simulink model "Real_Acrobot_Simulation"  (R2022b)
settings: Solver=ode23t  StartTime=0.0  StopTime=35  FixedStep=0.0002  MaxStep=1.6  RelTol=1e-4
values from neighbouring files (symbols this model uses):
  g = 9.81    [linearizalas.m]    (also in real_parameters.m)
  K = inv(R+B_d'*P*B_d)*B_d'*P*A_d    [DLQR.m]    (also in Main.m = LQR_function(A, B))
  l1 = 0.4    [real_parameters.m]
  m_weight = 0.086    [real_parameters.m]
  Q0 = [0.1 0 0 0]    [real_parameters.m]
undefined symbols (not defined in the file or in its folder): X, Y, Z
libraries: sm_lib x44, nesl_utility x22, fl_lib x15, simulink_extras x4, ee_lib x2, hdlsllib x1, eeQuadratureDecoder x1, slpidlib x1, simulink x1
(part 2 of 2)

== system Real_Acrobot_Simulation/Acrobot modelling/Joint 1/Encoder ==
  Electrical Reference : fl_lib/Electrical/Electrical Elements/Electrical Reference
  Incremental Shaft Encoder : ee_lib/Sensors & Transducers/Incremental Shaft Encoder  NPulse=600  Vm=5 V  angle0=0 deg
      settings: InternalSimscapePortConfiguration="{\"Bottom\":[],\"Left\":[{\"id\":\"R\",\"label\":\"R\",\"type\":\"foundation.mechanical.rotational.rotational\"},{\"id\":\"C\",\"label\":\"C\",\"type\":\"foundation.mechanical.rotational.rotational\"}],\"Right\":[{\"id\":\"A\",\"label\":\"A\",\"type\":\"foundation.electrical.electrical\"},{\"id\":\"B\",\"label\":\"B\",\"type\":\"foundation.electrical.electrical\"},{\"id\":\"Z\",\"label\":\"Z\",\"type\":\"foundation.electrical.electrical\"},{\"id\":\"GND\",\"label\":\"REF\",\"type\":\"foundation.electrical.electrical\"}],\"Top\":[]}"
  Mechanical Rotational Reference1 : fl_lib/Mechanical/Rotational Elements/Mechanical Rotational Reference
  PS-Simulink Converter : nesl_utility/PS-Simulink Converter  PhysicalDomain=network_engine_domain  SubClassName=ps_output  LeftPortType=input  RightPortType=output  PseudoPeriodic=off  Frequencies=[]  VectorFormat=1-D array  Unit=inherit  AffineConversion=off
  PS-Simulink Converter4 : nesl_utility/PS-Simulink Converter  PhysicalDomain=network_engine_domain  SubClassName=ps_output  LeftPortType=input  RightPortType=output  PseudoPeriodic=off  Frequencies=[]  VectorFormat=1-D array  Unit=inherit  AffineConversion=off
  Rotational Multibody Interface : fl_lib/Mechanical/Multibody Interfaces/Rotational Multibody Interface
  Voltage Sensor4 : fl_lib/Electrical/Electrical Sensors/Voltage Sensor
  Voltage Sensor5 : fl_lib/Electrical/Electrical Sensors/Voltage Sensor
  dq1 : PMIOPort  Side=Left
  B : Outport
  A : Outport  Port=2
  wires:
  PS-Simulink Converter/1 -> A/1
  PS-Simulink Converter4/1 -> B/1
  connections:
  Incremental Shaft Encoder/LConn1 -- Rotational Multibody Interface/RConn2
  Electrical Reference/LConn1 -- Incremental Shaft Encoder/RConn4 -- Voltage Sensor5/RConn2 -- Voltage Sensor4/RConn2
  dq1/RConn1 -- Rotational Multibody Interface/RConn1
  Mechanical Rotational Reference1/LConn1 -- Rotational Multibody Interface/LConn2 -- Incremental Shaft Encoder/LConn2
  Voltage Sensor4/LConn1 -- Incremental Shaft Encoder/RConn2
  Voltage Sensor5/LConn1 -- Incremental Shaft Encoder/RConn1
  Voltage Sensor4/RConn1 -- PS-Simulink Converter4/LConn1
  Voltage Sensor5/RConn1 -- PS-Simulink Converter/LConn1

== system Real_Acrobot_Simulation/Acrobot modelling/Joint 1/Revolute Join1 ==
  Joint1 : sm_lib/Joints/Revolute Joint  JointMode=Normal  SenseConstraintForce=off  SenseConstraintForceX=off  SenseConstraintForceY=off  SenseConstraintForceZ=off  SenseConstraintTorque=off  SenseConstraintTorqueX=off  SenseConstraintTorqueY=off  SenseConstraintTorqueZ=off  SenseTotalForce=off  SenseTotalForceX=off  SenseTotalForceY=off  SenseTotalForceZ=off  SenseTotalTorque=off  SenseTotalTorqueX=off  SenseTotalTorqueY=off  SenseTotalTorqueZ=off  CompositeWrenchDir=FollowerOnBase  CompositeWrenchFrame=BaseFrame  EquilibriumPosition=0  EquilibriumPositionUnits=deg  SpringStiffness=0  SpringStiffnessUnits=N*m/deg  DampingCoefficient=0.002  DampingCoefficientUnits=N*m/(rad/s)  TorqueActuationMode=NoTorque  MotionActuationMode=ComputedMotion  SensePosition=on  SenseVelocity=on  SenseAcceleration=off  SenseTorqueForce=off  SenseLowerLimitTorqueForce=off  SenseUpperLimitTorqueForce=off  LowerLimitSpecify=off  LowerLimitBound=-90  LowerLimitBoundUnits=deg  LowerLimitStiffness=1e4  LowerLimitStiffnessUnits=N*m/deg  LowerLimitDamping=10  LowerLimitDampingUnits=N*m/(deg/s)  LowerLimitTransitionRegionWidth=0.1  LowerLimitTransitionRegionWidthUnits=deg  UpperLimitSpecify=off  UpperLimitBound=90  UpperLimitBoundUnits=deg  UpperLimitStiffness=1e4  UpperLimitStiffnessUnits=N*m/deg  UpperLimitDamping=10  UpperLimitDampingUnits=N*m/(deg/s)  UpperLimitTransitionRegionWidth=0.1  UpperLimitTransitionRegionWidthUnits=deg  PositionTargetSpecify=on  PositionTargetPriority=High  PositionTargetValue=Q0(1)  PositionTargetValueUnits=rad  VelocityTargetSpecify=on  VelocityTargetPriority=High  VelocityTargetValue=Q0(2)  VelocityTargetValueUnits=rad/s
  PS-Simulink Converter2 : nesl_utility/PS-Simulink Converter  PhysicalDomain=network_engine_domain  SubClassName=ps_output  LeftPortType=input  RightPortType=output  PseudoPeriodic=off  Frequencies=[]  VectorFormat=1-D array  Unit=inherit  AffineConversion=off
  PS-Simulink Converter3 : nesl_utility/PS-Simulink Converter  PhysicalDomain=network_engine_domain  SubClassName=ps_output  LeftPortType=input  RightPortType=output  PseudoPeriodic=off  Frequencies=[]  VectorFormat=1-D array  Unit=inherit  AffineConversion=off
  Trans Z1 : sm_lib/Frames and Transforms/Rigid Transform  TranslationMethod=StandardAxis  TranslationStandardOffset=2  TranslationLengthUnit=cm  TranslationStandardAxis=+Z  TranslationCartesianOffset=[0 0 0]  TranslationROffset=0  TranslationROffsetUnits=m  TranslationZOffset=0  TranslationZOffsetUnits=m  TranslationThetaOffset=0  TranslationThetaOffsetUnits=deg  RotationMethod=None  RotationAngleUnits=deg  RotationStandardAxis=+X  RotationAngle=90  RotationArbitraryAxis=[0 0 1]  FollAlignAxisA=+X  BaseAlignAxisA=+Y  FollAlignAxisB=+Y  BaseAlignAxisB=+Z  RotationSequenceAxes=FollowerAxes  RotationSequence=XYX  RotationSequenceAngles=[0 0 0]  RotationSequenceAnglesUnits=deg  RotationMatrix=[1 0 0; 0 1 0; 0 0 1]  Quaternion=[1 0 0 0]
  " In" : PMIOPort  Side=Left
  dq1_mech : PMIOPort  Port=2  Side=Right
  Out : PMIOPort  Port=3  Side=Right
  q1 : Outport
  dq1 : Outport  Port=2
  wires:
  PS-Simulink Converter2/1 -> q1/1
  PS-Simulink Converter3/1 -> dq1/1
  connections:
  Trans Z1/RConn1 -- Joint1/LConn1
  Joint1/RConn1 -- Out/RConn1
  Trans Z1/LConn1 -- " In"/RConn1
  Joint1/RConn3 -- PS-Simulink Converter3/LConn1 -- dq1_mech/RConn1
  PS-Simulink Converter2/LConn1 -- Joint1/RConn2

== system Real_Acrobot_Simulation/Acrobot modelling/Joint 1/Wrap Angle ==
  In1 : Inport
  Add1 : Sum  Inputs=+-
  Bias : Bias  Bias=pi  SaturateOnIntegerOverflow=off
  Constant : Constant  Value=2*pi
  Constant2 : Constant  Value=2*pi
  Divide : Product  Inputs=*/
  Floor : Rounding
  Product : Product  Inputs=**
  q1 : Outport
  wires:
  Constant/1 -> Divide/2
  In1/1 -> Bias/1, Add1/1
  Divide/1 -> Floor/1
  Floor/1 -> Product/1
  Constant2/1 -> Product/2
  Product/1 -> Add1/2
  Add1/1 -> q1/1
  Bias/1 -> Divide/1

== system Real_Acrobot_Simulation/Acrobot modelling/Joint 1/Wrap Angle pi-pi ==
  In1 : Inport
  Add1 : Sum  Inputs=+-
  Bias : Bias  Bias=pi  SaturateOnIntegerOverflow=off
  Constant : Constant  Value=2*pi
  Constant2 : Constant  Value=2*pi
  Divide : Product  Inputs=*/
  Floor : Rounding
  Product : Product  Inputs=**
  q1 : Outport
  wires:
  Constant/1 -> Divide/2
  In1/1 -> Bias/1, Add1/1
  Divide/1 -> Floor/1
  Floor/1 -> Product/1
  Constant2/1 -> Product/2
  Product/1 -> Add1/2
  Add1/1 -> q1/1
  Bias/1 -> Divide/1

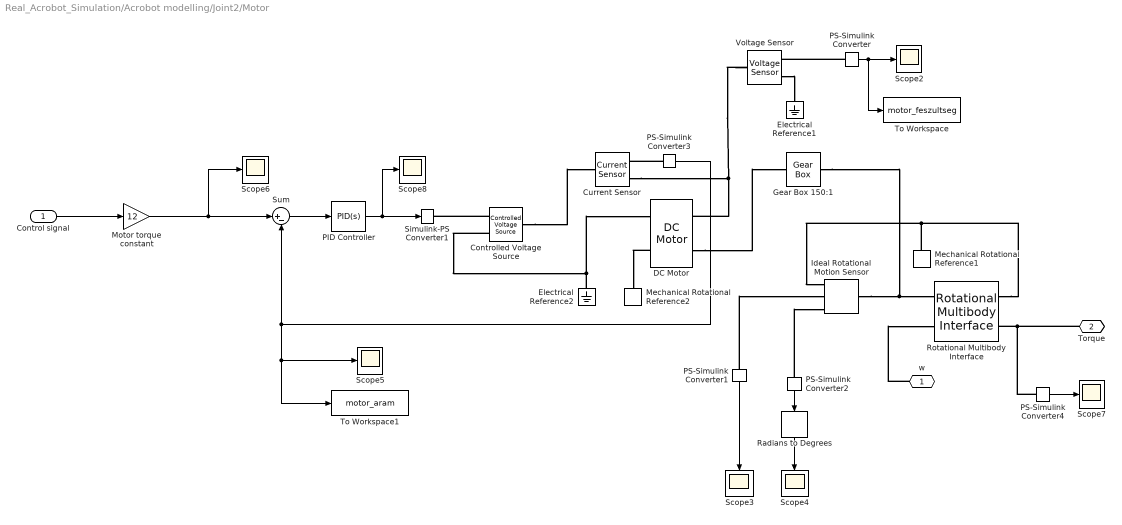
== system Real_Acrobot_Simulation/Acrobot modelling/Joint2/Motor ==
  Control signal : Inport
  Controlled Voltage Source : fl_lib/Electrical/Electrical Sources/Controlled Voltage Source
  Current Sensor : fl_lib/Electrical/Electrical Sensors/Current Sensor
  DC Motor : ee_lib/Electromechanical/Brushed Motors/DC Motor  field_option=ee.enum.field_option.pm  Rf=100 Ohm  Lf=1 H  Laf=0.15 H  If0=0 A  parameterization=ee.enum.dcparam_option.circuit_param  Ra=3.9 Ohm  La=12e-6 H  emf_or_torque=ee.enum.emf_or_torque.kv  Kv=0.072e-3 V/rpm  Ki=6.876e-4 N*m/A  T_stall=0.24e-3 N*m  w_max=19100 rpm  w_rated=15000 rpm  P_rated=0.08 W  V_rated=1.5 V  lam_param=ee.enum.lam_param.damping  i_noload=0 A  V_i_noload=1.5 V  J=0.01 cm^2*g  lam=0 N*m*s/rad  speed0=0 rpm  enable_fault_armature=simscape.enum.onoff.off  rev_faulted=1 / 3  G_faulted_armature=1e-5 S  fault_trigger_armature=ee.enum.faults.faultTrigger.temporal  t_fault_armature=1 s  max_permissible_current_armature=inf A  t_fail_on_current_armature=1 s  enable_fault_field=simscape.enum.onoff.off  G_faulted_field=1e-5 S  fault_trigger_field=ee.enum.faults.faultTrigger.temporal  t_fault_field=1 s  max_permissible_current_field=inf A  t_fail_on_current_field=1 s  fault_action=simscape.enum.assert.action.none  alpha=3.93e-3 1/K  Tmeas=25 degC  thermal_mass=100 J/K  initial_temperature=25 degC
  Electrical Reference1 : fl_lib/Electrical/Electrical Elements/Electrical Reference
  Electrical Reference2 : fl_lib/Electrical/Electrical Elements/Electrical Reference
  Gear Box 150:1 : fl_lib/Mechanical/Mechanisms/Gear Box  ratio=150  t_in_specify=off  t_in_priority=None  t_in=0 N*m  t_in_nominal_specify=off  t_in_nominal_unit=N*m  t_in_nominal_value=1  t_out_specify=off  t_out_priority=None  t_out=0 N*m  t_out_nominal_specify=off  t_out_nominal_unit=N*m  t_out_nominal_value=1
  Ideal Rotational Motion Sensor : fl_lib/Mechanical/Mechanical Sensors/Ideal Rotational Motion Sensor  reference=foundation.enum.MeasurementReference.difference  acceleration_port=false  velocity_port=true  position_port=true  wrap_angle=false  offset=0 rad
  Mechanical Rotational Reference1 : fl_lib/Mechanical/Rotational Elements/Mechanical Rotational Reference
  Mechanical Rotational Reference2 : fl_lib/Mechanical/Rotational Elements/Mechanical Rotational Reference
  Motor torque constant : Gain  Gain=12
  PID Controller : slpidlib/PID Controller  Controller=PID  Form=Parallel  TimeDomain=Continuous-time  UseExternalTs=off  SampleTime=-1  IntegratorMethod=Forward Euler  FilterMethod=Forward Euler  ControllerParametersSource=internal  P=10  I=0.1  UseKiTs=off  D=0.5  N=100  UseFilter=on  TunerSelectOption=Transfer Function Based (PID Tuner App)  InitialConditionSource=internal  InitialConditionForIntegrator=0  InitialConditionForFilter=0  DifferentiatorICPrevScaledInput=0  ExternalReset=none  TrackingMode=off  Kt=1  LimitOutput=off  SatLimitsSource=internal  UpperSaturationLimit=inf  LowerSaturationLimit=-inf  LinearizeAsGain=on  AntiWindupMode=none  Kb=1  LimitIntegrator=off  UpperIntegratorSaturationLimit=inf  LowerIntegratorSaturationLimit=-inf  POutMin=[]  POutMax=[]  IOutMin=[]  IOutMax=[]  DOutMin=[]  DOutMax=[]  NOutMin=[]  NOutMax=[]  SumOutMin=[]  SumOutMax=[]  SaturationOutMin=[]  SaturationOutMax=[]  PParamMin=[]  PParamMax=[]  IParamMin=[]  IParamMax=[]  DParamMin=[]  DParamMax=[]  NParamMin=[]  NParamMax=[]  KbParamMin=[]  KbParamMax=[]  KtParamMin=[]  KtParamMax=[]  KbOutMin=[]  KbOutMax=[]  KtOutMin=[]  KtOutMax=[]  IntegratorOutMin=[]  IntegratorOutMax=[]  FilterOutMin=[]  FilterOutMax=[]  SumI1OutMin=[]  SumI1OutMax=[]  SumI2OutMin=[]  SumI2OutMax=[]  SumI3OutMin=[]  SumI3OutMax=[]  SumI4OutMin=[]  SumI4OutMax=[]  SumDOutMin=[]  SumDOutMax=[]  DifferentiatorOutMin=[]  DifferentiatorOutMax=[]  FilterDiffOutCoefMin=[]  FilterDiffOutCoefMax=[]  ReciprocalOutMin=[]  ReciprocalOutMax=[]  SumDenOutMin=[]  SumDenOutMax=[]  SumNumOutMin=[]  SumNumOutMax=[]  DivideOutMin=[]  DivideOutMax=[]  UdiffTsProdOutMin=[]  UdiffTsProdOutMax=[]  NTsProdOutMin=[]  NTsProdOutMax=[]  UintegralTsProdOutMin=[]  UintegralTsProdOutMax=[]  UngainTsProdOutMin=[]  UngainTsProdOutMax=[]  ClampingZeroOutDataTypeStr=Inherit: Inherit via back propagation  ClampingZeroOutMin=[]  ClampingZeroOutMax=[]  FilterDenConstantOutDataTypeStr=Inherit: Inherit via back propagation  FilterDenConstantOutMin=[]  FilterDenConstantOutMax=[]  PCopyOutDataTypeStr=Inherit: Inherit via back propagation  PCopyOutMin=[]  PCopyOutMax=[]  NCopyOutDataTypeStr=Inherit: Inherit via back propagation  NCopyOutMin=[]  NCopyOutMax=[]  IntegratorContinuousStateAttributes=''  IntegratorStateMustResolveToSignalObject=off  IntegratorRTWStateStorageClass=Auto  FilterContinuousStateAttributes=''  FilterStateMustResolveToSignalObject=off  FilterRTWStateStorageClass=Auto  ParallelPVariant=InternalParameters  IdealPVariant=Disabled  IVariant=InternalParameters  DVariant=InternalParameters  IntegratorVariant=Continuous  SatVariant=Disabled  AWVariant=Passthrough  PCopyVariant=Disabled  TRVariant=Disabled  FdbkBlocksVariant=Forward  IdealPFdbkVariant=Disabled  SatFdbkVariant=Disabled  DerivativeFilterVariant=ContFilter  NVariant=InternalParameters  NCopyVariant=Disabled  FilterICVariant=InternalICsFilter  IntegratorICVariant=InternalICs  ExternalResetVariant=Disabled  TRSumVariant=Passthrough  SumFdbkVariant=Disabled  SumVariant=Sum_PID  TsampFilterVariant=InternalTs  TsampNgainVariant=Passthrough  TsampIntegralVariant=Passthrough  ExternalSaturationOutDataTypeStr=Inherit: Same as second input
  PS-Simulink Converter{,1..2,4} (4 alike) : nesl_utility/PS-Simulink Converter  PhysicalDomain=network_engine_domain  SubClassName=ps_output  LeftPortType=input  RightPortType=output  PseudoPeriodic=off  Frequencies=[]  VectorFormat=1-D array  Unit=inherit  AffineConversion=off
  PS-Simulink Converter3 : nesl_utility/PS-Simulink Converter  PhysicalDomain=network_engine_domain  SubClassName=ps_output  LeftPortType=input  RightPortType=output  PseudoPeriodic=off  Frequencies=[]  VectorFormat=inherit  Unit=inherit  AffineConversion=off
  Radians to Degrees : simulink_extras/Transformations/Radians to Degrees
  Rotational Multibody Interface : fl_lib/Mechanical/Multibody Interfaces/Rotational Multibody Interface
  Scope{2..8} (7 alike) : Scope
  Simulink-PS Converter1 : nesl_utility/Simulink-PS Converter  PhysicalDomain=network_engine_domain  SubClassName=ps_input  LeftPortType=input  RightPortType=output  PseudoPeriodic=off  Frequencies=[]  NoiseDistribution=none  NoiseParameters=[]  Unit=1  AffineConversion=off  FilteringAndDerivatives=provide  SimscapeFilterOrder=1  InputFilterTimeConstant=0.001  UdotUserProvided=0
  Sum : Sum  Inputs=|+-
  To Workspace : ToWorkspace  VariableName=motor_feszultseg  SaveFormat=Timeseries  SampleTime=-1
  To Workspace1 : ToWorkspace  VariableName=motor_aram  SaveFormat=Timeseries  SampleTime=-1
  Voltage Sensor : fl_lib/Electrical/Electrical Sensors/Voltage Sensor
  w : PMIOPort  Side=Left
  Torque : PMIOPort  Port=2  Side=Right
  wires:
  PS-Simulink Converter/1 -> To Workspace/1, Scope2/1
  PS-Simulink Converter2/1 -> Radians to Degrees/1
  Radians to Degrees/1 -> Scope4/1
  PS-Simulink Converter1/1 -> Scope3/1
  Control signal/1 -> Motor torque constant/1
  Motor torque constant/1 -> Scope6/1, Sum/1
  PS-Simulink Converter3/1 -> Sum/2, Scope5/1, To Workspace1/1
  PS-Simulink Converter4/1 -> Scope7/1
  Sum/1 -> PID Controller/1
  PID Controller/1 -> Simulink-PS Converter1/1, Scope8/1
  connections:
  PS-Simulink Converter/LConn1 -- Voltage Sensor/RConn1
  Mechanical Rotational Reference1/LConn1 -- Ideal Rotational Motion Sensor/RConn1 -- Rotational Multibody Interface/LConn2
  Ideal Rotational Motion Sensor/LConn1 -- Gear Box 150:1/RConn1 -- Rotational Multibody Interface/RConn2
  PS-Simulink Converter1/LConn1 -- Ideal Rotational Motion Sensor/RConn2
  PS-Simulink Converter2/LConn1 -- Ideal Rotational Motion Sensor/RConn3
  Voltage Sensor/RConn2 -- Electrical Reference1/LConn1
  Torque/RConn1 -- PS-Simulink Converter4/LConn1 -- Rotational Multibody Interface/LConn1
  DC Motor/RConn2 -- Mechanical Rotational Reference2/LConn1
  PS-Simulink Converter3/LConn1 -- Current Sensor/RConn1
  Electrical Reference2/LConn1 -- DC Motor/RConn1 -- Controlled Voltage Source/RConn2
  Current Sensor/RConn2 -- Voltage Sensor/LConn1 -- DC Motor/LConn1
  DC Motor/LConn2 -- Gear Box 150:1/LConn1
  w/RConn1 -- Rotational Multibody Interface/RConn1
  Controlled Voltage Source/LConn1 -- Current Sensor/LConn1
  Controlled Voltage Source/RConn1 -- Simulink-PS Converter1/RConn1

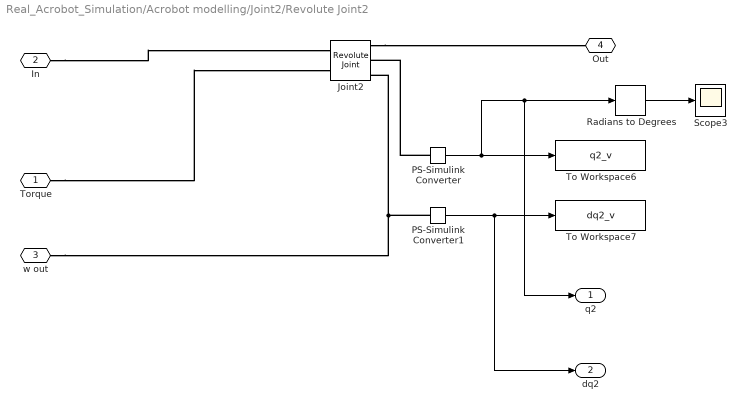
== system Real_Acrobot_Simulation/Acrobot modelling/Joint2/Revolute Joint2 ==
  Joint2 : sm_lib/Joints/Revolute Joint  JointMode=Normal  SenseConstraintForce=off  SenseConstraintForceX=off  SenseConstraintForceY=off  SenseConstraintForceZ=off  SenseConstraintTorque=off  SenseConstraintTorqueX=off  SenseConstraintTorqueY=off  SenseConstraintTorqueZ=off  SenseTotalForce=off  SenseTotalForceX=off  SenseTotalForceY=off  SenseTotalForceZ=off  SenseTotalTorque=off  SenseTotalTorqueX=off  SenseTotalTorqueY=off  SenseTotalTorqueZ=off  CompositeWrenchDir=FollowerOnBase  CompositeWrenchFrame=BaseFrame  EquilibriumPosition=0  EquilibriumPositionUnits=deg  SpringStiffness=0  SpringStiffnessUnits=N*m/deg  DampingCoefficient=0  DampingCoefficientUnits=N*m/(deg/s)  TorqueActuationMode=InputTorque  MotionActuationMode=ComputedMotion  SensePosition=on  SenseVelocity=on  SenseAcceleration=off  SenseTorqueForce=off  SenseLowerLimitTorqueForce=off  SenseUpperLimitTorqueForce=off  LowerLimitSpecify=on  LowerLimitBound=-90  LowerLimitBoundUnits=deg  LowerLimitStiffness=1e4  LowerLimitStiffnessUnits=N*m/deg  LowerLimitDamping=10  LowerLimitDampingUnits=N*m/(deg/s)  LowerLimitTransitionRegionWidth=0.1  LowerLimitTransitionRegionWidthUnits=deg  UpperLimitSpecify=on  UpperLimitBound=90  UpperLimitBoundUnits=deg  UpperLimitStiffness=1e4  UpperLimitStiffnessUnits=N*m/deg  UpperLimitDamping=10  UpperLimitDampingUnits=N*m/(deg/s)  UpperLimitTransitionRegionWidth=0.1  UpperLimitTransitionRegionWidthUnits=deg  PositionTargetSpecify=on  PositionTargetPriority=High  PositionTargetValue=Q0(3)  PositionTargetValueUnits=rad  VelocityTargetSpecify=on  VelocityTargetPriority=High  VelocityTargetValue=Q0(4)  VelocityTargetValueUnits=rad/s
  PS-Simulink Converter : nesl_utility/PS-Simulink Converter  PhysicalDomain=network_engine_domain  SubClassName=ps_output  LeftPortType=input  RightPortType=output  PseudoPeriodic=off  Frequencies=[]  VectorFormat=1-D array  Unit=inherit  AffineConversion=off
  PS-Simulink Converter1 : nesl_utility/PS-Simulink Converter  PhysicalDomain=network_engine_domain  SubClassName=ps_output  LeftPortType=input  RightPortType=output  PseudoPeriodic=off  Frequencies=[]  VectorFormat=1-D array  Unit=inherit  AffineConversion=off
  Radians to Degrees : simulink_extras/Transformations/Radians to Degrees
  Scope3 : Scope
  To Workspace6 : ToWorkspace  VariableName=q2_v  SaveFormat=Timeseries  SampleTime=-1
  To Workspace7 : ToWorkspace  VariableName=dq2_v  SaveFormat=Timeseries  SampleTime=-1
  Torque : PMIOPort  Side=Left
  In : PMIOPort  Port=2  Side=Left
  w out : PMIOPort  Port=3  Side=Right
  Out : PMIOPort  Port=4  Side=Right
  q2 : Outport
  dq2 : Outport  Port=2
  wires:
  PS-Simulink Converter1/1 -> dq2/1, To Workspace7/1
  PS-Simulink Converter/1 -> Radians to Degrees/1, q2/1, To Workspace6/1
  Radians to Degrees/1 -> Scope3/1
  connections:
  PS-Simulink Converter/LConn1 -- Joint2/RConn2
  PS-Simulink Converter1/LConn1 -- Joint2/RConn3 -- w out/RConn1
  In/RConn1 -- Joint2/LConn1
  Joint2/RConn1 -- Out/RConn1
  Torque/RConn1 -- Joint2/LConn2

== system Real_Acrobot_Simulation/Acrobot modelling/Controller/Controller/LQR Control ==
  note: Balancing - linearizalt rendszerre
  note: -pi eltolas
      | A linearizalt szabalyozashoz csak
      | itt meg akar modulot probalgatni
  note: q1 q2 dq1 dq2
  note: q1 q2 dq1 dq2
  States : Inport
  Bias : Bias  Bias=-pi  SaturateOnIntegerOverflow=off
  Demux1 : Demux
  Gain : Gain  Gain=-K  Multiplication=Matrix(K*u)
  Mux1 : Mux
  Scope1 : Scope
  Scope2 : Scope
  Wrap Angle pi-pi : Subsystem
  Control signal : Outport
  wires:
  Mux1/1 -> Gain/1, Scope1/1
  States/1 -> Demux1/1
  Demux1/1 -> Bias/1
  Demux1/4 -> Mux1/4
  Demux1/2 -> Mux1/2
  Demux1/3 -> Mux1/3
  Bias/1 -> Wrap Angle pi-pi/1(In1)
  Wrap Angle pi-pi/1(q1) -> Mux1/1
  Gain/1 -> Control signal/1, Scope2/1

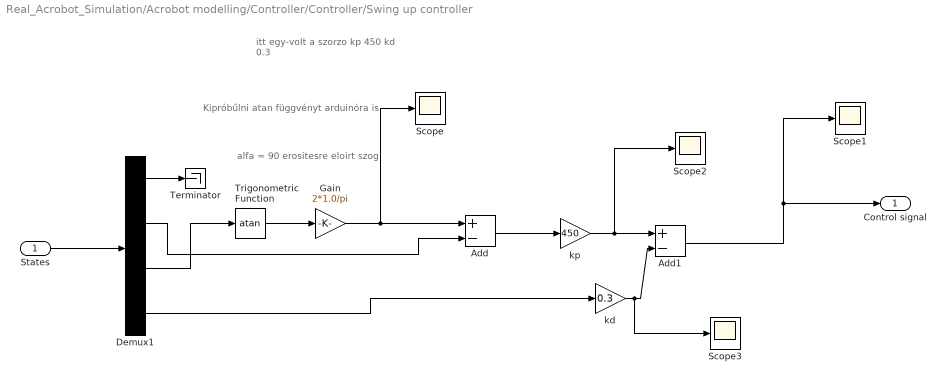
== system Real_Acrobot_Simulation/Acrobot modelling/Controller/Controller/Swing up controller ==
  note: itt egy-volt a szorzo
      | kp 450
      | kd 0.3
  note: Kipróbűlni atan függvényt arduinóra is
  note: alfa = 90 erositesre eloirt szog
  States : Inport
  Add : Sum  Inputs=+-
  Add1 : Sum  Inputs=+-
  Demux1 : Demux
  Gain : Gain  Gain=2*1.0/pi
  Scope{,1..3} (4 alike) : Scope
  Terminator : Terminator
  Trigonometric Function : Trigonometry  Operator=atan
  kd : Gain  Gain=0.3
  kp : Gain  Gain=450
  Control signal : Outport
  wires:
  States/1 -> Demux1/1
  Trigonometric Function/1 -> Gain/1
  Gain/1 -> Add/1, Scope/1
  kd/1 -> Scope3/1, Add1/2
  Demux1/4 -> kd/1
  Add1/1 -> Scope1/1, Control signal/1
  Demux1/1 -> Terminator/1
  Demux1/3 -> Trigonometric Function/1
  Demux1/2 -> Add/2
  Add/1 -> kp/1
  kp/1 -> Add1/1, Scope2/1

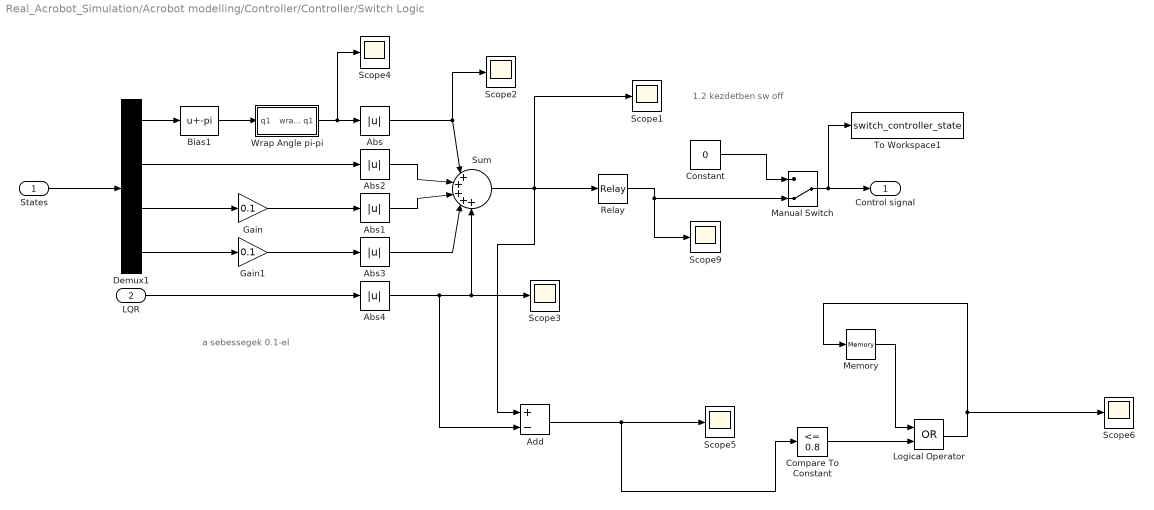
== system Real_Acrobot_Simulation/Acrobot modelling/Controller/Controller/Switch Logic ==
  note: a sebessegek 0.1-el
  note: 1.2 kezdetben sw off
  States : Inport
  LQR : Inport  Port=2
  Abs{,1..4} (5 alike) : Abs  SaturateOnIntegerOverflow=off
  Add : Sum  Inputs=+-
  Bias1 : Bias  Bias=-pi  SaturateOnIntegerOverflow=off
  Compare To Constant : hdlsllib/Logic and Bit Operations/Compare To Constant  relop=<=  const=0.8  OutDataTypeStr=boolean
  Constant : Constant  Value=0
  Demux1 : Demux
  Gain : Gain  Gain=0.1
  Gain1 : Gain  Gain=0.1
  Logical Operator : Logic  Operator=OR  AllPortsSameDT=off  OutDataTypeStr=boolean
  Manual Switch : ManualSwitch  CurrentSetting=0
  Memory : Memory
  Relay : Relay  OnSwitchValue=50  OffSwitchValue=1.2  OnOutputValue=0  OffOutputValue=1
  Scope{1..6,9} (7 alike) : Scope
  Sum : Sum  Inputs=|+++++
  To Workspace1 : ToWorkspace  VariableName=switch_controller_state  SaveFormat=Timeseries  SampleTime=-1
  Wrap Angle pi-pi : Subsystem
  Control signal : Outport
  wires:
  States/1 -> Demux1/1
  Demux1/2 -> Abs2/1
  Demux1/4 -> Gain1/1
  Demux1/3 -> Gain/1
  Gain1/1 -> Abs3/1
  Abs2/1 -> Sum/2
  Abs3/1 -> Sum/4
  Sum/1 -> Relay/1, Scope1/1, Add/1
  Abs/1 -> Scope2/1, Sum/1
  Gain/1 -> Abs1/1
  Abs1/1 -> Sum/3
  Demux1/1 -> Bias1/1
  Bias1/1 -> Wrap Angle pi-pi/1(q1)
  Wrap Angle pi-pi/1(wrapped q1) -> Abs/1, Scope4/1
  Relay/1 -> Manual Switch/2, Scope9/1
  Manual Switch/1 -> To Workspace1/1, Control signal/1
  Constant/1 -> Manual Switch/1
  LQR/1 -> Abs4/1
  Abs4/1 -> Add/2, Scope3/1, Sum/5
  Add/1 -> Compare To Constant/1, Scope5/1
  Memory/1 -> Logical Operator/1
  Logical Operator/1 -> Memory/1, Scope6/1
  Compare To Constant/1 -> Logical Operator/2

== system Real_Acrobot_Simulation/Acrobot modelling/Controller/Controller/LQR Control/Wrap Angle pi-pi ==
  In1 : Inport
  Add1 : Sum  Inputs=+-
  Bias : Bias  Bias=pi  SaturateOnIntegerOverflow=off
  Constant : Constant  Value=2*pi
  Constant2 : Constant  Value=2*pi
  Divide : Product  Inputs=*/
  Floor : Rounding
  Product : Product  Inputs=**
  q1 : Outport
  wires:
  Constant/1 -> Divide/2
  In1/1 -> Bias/1, Add1/1
  Divide/1 -> Floor/1
  Floor/1 -> Product/1
  Constant2/1 -> Product/2
  Product/1 -> Add1/2
  Add1/1 -> q1/1
  Bias/1 -> Divide/1

== system Real_Acrobot_Simulation/Acrobot modelling/Controller/Controller/Switch Logic/Wrap Angle pi-pi ==
  q1 : Inport
  Add1 : Sum  Inputs=+-
  Bias : Bias  Bias=pi  SaturateOnIntegerOverflow=off
  Constant : Constant  Value=2*pi
  Constant2 : Constant  Value=2*pi
  Divide : Product  Inputs=*/
  Floor : Rounding
  Product : Product  Inputs=**
  wrapped q1 : Outport
  wires:
  Constant/1 -> Divide/2
  q1/1 -> Bias/1, Add1/1
  Divide/1 -> Floor/1
  Floor/1 -> Product/1
  Constant2/1 -> Product/2
  Product/1 -> Add1/2
  Add1/1 -> wrapped q1/1
  Bias/1 -> Divide/1

== matlab function Real_Acrobot_Simulation/Acrobot modelling/MATLAB Function ==
  data: q1 input; dq1 input; q2 input; dq2 input; E output; E_Et output
function [E,E_Et] = Energy(q1,dq1,q2,dq2)

g = 9.81;

m1 = 0.1012;
m2 = 0.1203;
l1 = 0.4;
l2 = 0.425;
lc1 = 0.2885;
lc2 = 0.34;
J1 = 0.0015;
J2 = 0.0018;

alfa1 = m1*lc1^2+m2*l1^2+J1;
alfa2 = m2*lc2^2+J2;
alfa3 = m2*l1*lc2;
beta1 = (m1*lc1 + m2*l1)*g;
beta2 = m2*lc2*g;

delta = alfa1*alfa2-alfa3^2*(cos(q2))^2;

m11 = alfa1 + alfa2 +2*alfa3*cos(q2);
m12 = alfa2+alfa3*cos(q2);
m21 = m12;
m22 = alfa2;

M = [m11 m12; m21 m22];

h1 = alfa3*(-2*dq1*dq2 - dq2^2)*sin(q2);
h2 = alfa3*dq1^2*sin(q2);

g1 = beta1*cos(q1) + beta2*cos(q1+q2);
g2 = beta2*cos(q1+q2);

kv = 66.3;
kD = 35.8;
kP = 61.2;

P = beta1*sin(q1-pi/2) + beta2*sin(q1-pi/2+q2);
E = (1/2)*[dq1 dq2]*M*[dq1 dq2]' + P;
% Target energy
Et = beta1+beta2;
E_Et = E-Et;

%tau = -(((kv*dq2+kP*q2)*delta+kD*(m21*(h1+g1)-m11*(h2+g2)))/(kD*m11+(E-Er)*delta));


end
